simulink model "SAD_project"  (R2023b)
settings: Solver=ode4  StartTime=t0  StopTime=tf  FixedStep=t_step  RelTol=1e-3
values from neighbouring files (symbols this model uses):
  A = 1e-2.*[6, 6, 6, 6, 4, 4, 12, 12, 12, 12]'    [SAD_project_code.m]
  A1 = ones(length(BODY),1)    [SAD_project_code.m]
  BODY = [1, 0, 0 ... (first row only)    [SAD_project_code.m]
  c = 3e8    (= 300000000)    [SAD_project_code.m]
  DCM_eci_per = rotationMatrix(rad2deg(i),rad2deg(OM), rad2deg(om))    [SAD_project_code.m]
  e = 0.001    [SAD_project_code.m]
  epsilon = deg2rad(23.45)    [SAD_project_code.m]
  Fe = 1358    [SAD_project_code.m]
  FS = 800e-9    (= 8e-07)    [SAD_project_code.m]
  H0 = 1e-9.*[-29404.8 -1450.9 4652.5]'    [SAD_project_code.m]
  i = deg2rad(60)    [SAD_project_code.m]
  I = [Ix, 0, 0; 0, Iy, 0; 0, 0, Iz]    [SAD_project_code.m]
  I_inv = inv(I)    [SAD_project_code.m]
  inc_tot = sqrt(inc_lin^2 + inc_acc^2)    [SAD_project_code.m]
  j_b = [0.01 0.05 0.01]'    [SAD_project_code.m]
  MJD2000_initial = date2mjd2000(date0)    [SAD_project_code.m]
  mu_E = astroConstants(13)    [SAD_project_code.m]
  n_e = sqrt(mu_E/a^3)    [SAD_project_code.m]
  p = a*(1-e^2)    [SAD_project_code.m]
  pd = 0.1.*A1    [SAD_project_code.m]
  ps = [0.5, 0.5, 0.5, 0.5, 0.5, 0.5, 0.1, 0.1, 0.1, 0.1]'    [SAD_project_code.m]
  q0 = [0 0 0 1]    [SAD_project_code.m]
  r1 = r(:,1) + CMC_position(1).*ones(10,1)    [SAD_project_code.m]
  r2 = r(:,2) + CMC_position(2).*ones(10,1)    [SAD_project_code.m]
  r3 = r(:,3)+ CMC_position(3).*ones(10,1)    [SAD_project_code.m]
  R_E = astroConstants(23)    [SAD_project_code.m]
  th0 = deg2rad(0)    [SAD_project_code.m]
  ts_sensor = t_step    (= 0.01)    [SAD_project_code.m]
  w0 = [wx0 wy0 wz0]'    [SAD_project_code.m]
  w_E = deg2rad(15.04)/60/60    [SAD_project_code.m]
  w_r = 0    [SAD_project_code.m]
libraries: matrix_library x6, simulink x1
settings Model: Creator=samue  LastModifiedBy=samue

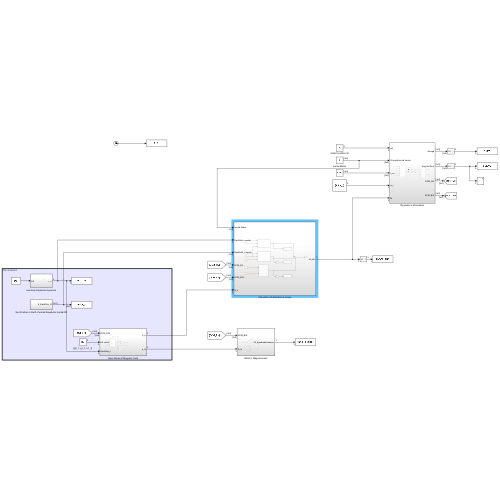
[thumbnail: Simulink's stored preview of the top-level diagram]
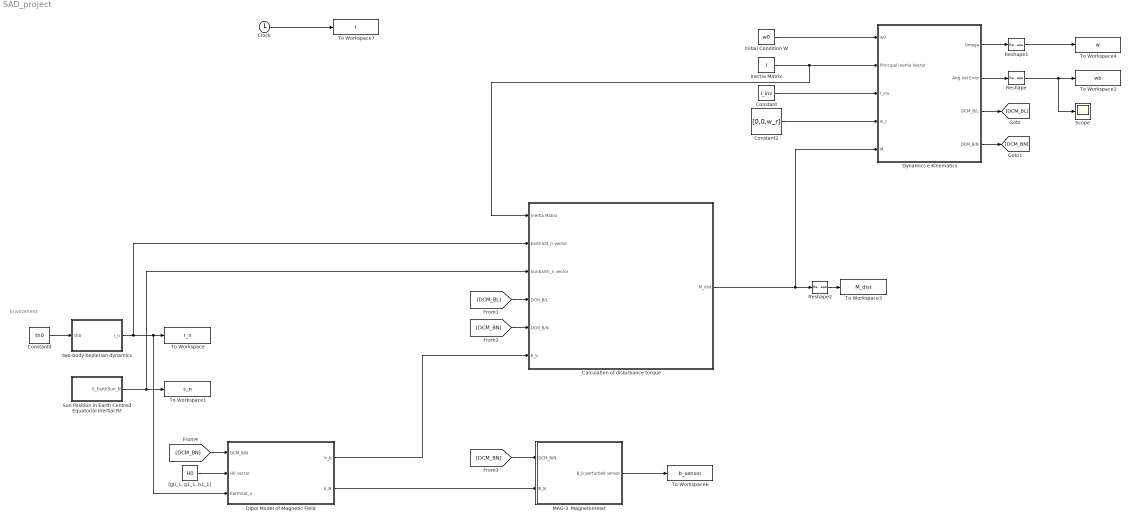
== system SAD_project ==
  note: Enviroment
  Calculation of disturbance torque : Subsystem
  Clock : Clock
  Constant : Constant  Value=I_inv
  Constant2 : Constant  Value=[0,0,w_r]
  Constant4 : Constant  Value=th0
  Dipol Model of Magnetic Field : Subsystem
  Dynamics e Kinematics : Subsystem
  Inertia Matrix : Constant  Value=I  VectorParams1D=off
  Initial Condition W : Constant  Value=w0
  MAG-3  Magnetometer : Subsystem
  Reshape : Reshape
  Reshape1 : Reshape
  Reshape2 : Reshape
  Scope : Scope
  Sun Position in Earth Centred Equatorial Inertial RF : Subsystem
  To Workspace : ToWorkspace  VariableName=r_n  SampleTime=-1
  To Workspace1 : ToWorkspace  VariableName=s_n  SampleTime=-1
  To Workspace2 : ToWorkspace  VariableName=wb  SampleTime=-1
  To Workspace3 : ToWorkspace  VariableName=M_dist  SaveFormat=Timeseries  SampleTime=-1
  To Workspace4 : ToWorkspace  VariableName=w  SampleTime=-1
  To Workspace6 : ToWorkspace  VariableName=b_sensor  SampleTime=-1
  To Workspace7 : ToWorkspace  VariableName=t  SampleTime=-1
  "[g0_1, g1_1, h1_1]" : Constant  Value=H0
  two-body Keplerian dynamics : Subsystem
  wires:
  two-body Keplerian dynamics/1(r_n) -> Calculation of disturbance torque/2(EarthSat_n vector), To Workspace/1, Dipol Model of Magnetic Field/3(EarthSat_n)
  Inertia Matrix/1 -> Calculation of disturbance torque/1(Inertia Matrix), Dynamics e Kinematics/2("Principal Inertia Vector ")
  Initial Condition W/1 -> Dynamics e Kinematics/1(w0)
  Reshape/1 -> Scope/1, To Workspace2/1
  Dynamics e Kinematics/2(Ang Vel Error) -> Reshape/1
  Dynamics e Kinematics/3(DCM_B/L) -> [DCM_BL]
  Dynamics e Kinematics/1(Omega) -> Reshape1/1
  Sun Position in Earth Centred Equatorial Inertial RF/1(S_EarthSun_N) -> To Workspace1/1, Calculation of disturbance torque/3(SunEarth_n vector)
  Constant2/1 -> Dynamics e Kinematics/4(w_r)
  Constant4/1 -> two-body Keplerian dynamics/1(th0)
  Constant/1 -> Dynamics e Kinematics/3(I_inv)
  Clock/1 -> To Workspace7/1
  Dynamics e Kinematics/4(DCM_B/N) -> [DCM_BN]
  Calculation of disturbance torque/1(M_dist) -> Reshape2/1, Dynamics e Kinematics/5(M)
  "[g0_1, g1_1, h1_1]"/1 -> Dipol Model of Magnetic Field/2(H0 vector)
  Dipol Model of Magnetic Field/1(b_b) -> Calculation of disturbance torque/6(B_b)
  MAG-3  Magnetometer/1(B_b perturbed sensor) -> To Workspace6/1
  [DCM_BN] -> MAG-3  Magnetometer/1(DCM_B/N)
  [DCM_BL] -> Calculation of disturbance torque/4(DCM_B/L)
  [DCM_BN] -> Calculation of disturbance torque/5(DCM_B/N)
  [DCM_BN] -> Dipol Model of Magnetic Field/1(DCM_B/N)
  Dipol Model of Magnetic Field/2(b_N) -> MAG-3  Magnetometer/2(B_N)
  Reshape1/1 -> To Workspace4/1
  Reshape2/1 -> To Workspace3/1

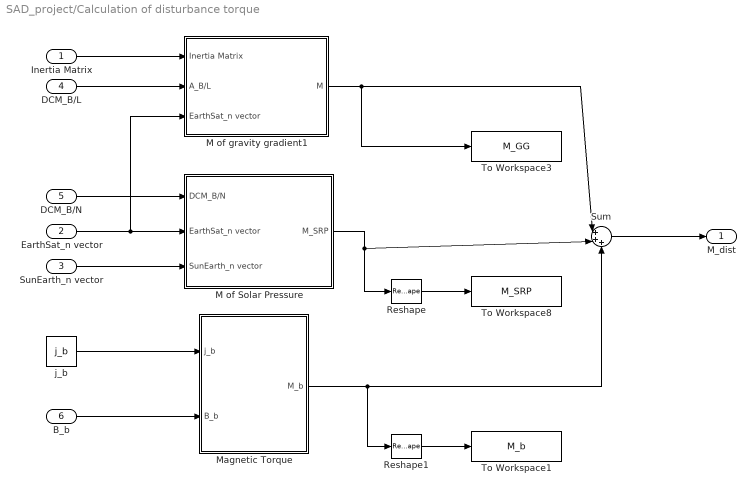
== system SAD_project/Calculation of disturbance torque ==
  Inertia Matrix : Inport
  EarthSat_n vector : Inport  Port=2
  SunEarth_n vector : Inport  Port=3
  DCM_B/L : Inport  Port=4
  DCM_B/N : Inport  Port=5
  B_b : Inport  Port=6
  M of Solar Pressure : Subsystem
  M of gravity gradient1 : Subsystem
  Magnetic Torque : Subsystem
  Reshape : Reshape
  Reshape1 : Reshape
  Sum : Sum  Inputs=|+++
  To Workspace1 : ToWorkspace  VariableName=M_b  SampleTime=-1
  To Workspace3 : ToWorkspace  VariableName=M_GG  SampleTime=-1
  To Workspace8 : ToWorkspace  VariableName=M_SRP  SampleTime=-1
  j_b : Constant  Value=j_b
  M_dist : Outport
  wires:
  DCM_B/L/1 -> M of gravity gradient1/2(A_B/L)
  j_b/1 -> Magnetic Torque/1(j_b)
  Magnetic Torque/1(M_b) -> Sum/3, Reshape1/1
  B_b/1 -> Magnetic Torque/2(B_b)
  Inertia Matrix/1 -> M of gravity gradient1/1(Inertia Matrix)
  M of Solar Pressure/1(M_SRP) -> Sum/2, Reshape/1
  EarthSat_n vector/1 -> M of gravity gradient1/3(EarthSat_n vector), M of Solar Pressure/2(EarthSat_n vector)
  DCM_B/N/1 -> M of Solar Pressure/1(DCM_B/N)
  SunEarth_n vector/1 -> M of Solar Pressure/3(SunEarth_n vector)
  Sum/1 -> M_dist/1
  Reshape/1 -> To Workspace8/1
  Reshape1/1 -> To Workspace1/1
  M of gravity gradient1/1(M) -> To Workspace3/1, Sum/1

== system SAD_project/Dipol Model of Magnetic Field ==
  note: CODE TO ADD
      | % Definition of Magnetic Field (Dipole model)
      |  j_b = [0.01 0.05 0.01]';
      | H0 = 1e-9.*[-29404.8 -1450.9 4652.5]';
  DCM_B/N : Inport
  H0 vector : Inport  Port=2
  EarthSat_n : Inport  Port=3
  Calculation of b_n : Subsystem
  Matrix Multiply : Product  Multiplication=Matrix(*)
  To Workspace : ToWorkspace  VariableName=bn  SampleTime=-1
  b_b : Outport
  b_N : Outport  Port=2
  wires:
  Matrix Multiply/1 -> b_b/1
  DCM_B/N/1 -> Matrix Multiply/1
  H0 vector/1 -> Calculation of b_n/1(H0 vector)
  EarthSat_n/1 -> Calculation of b_n/2(EarthSat_n)
  Calculation of b_n/1(b_N) -> To Workspace/1, b_N/1, Matrix Multiply/2

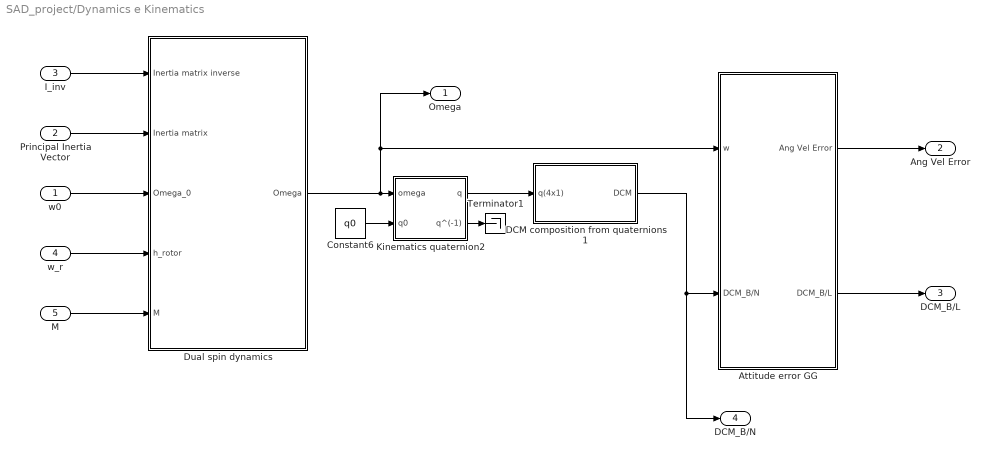
== system SAD_project/Dynamics e Kinematics ==
  w0 : Inport
  "Principal Inertia Vector " : Inport  Port=2
  I_inv : Inport  Port=3
  w_r : Inport  Port=4
  M : Inport  Port=5
  Attitude error GG : Subsystem
  Constant6 : Constant  Value=q0
  DCM composition from quaternions 1 : Subsystem  AncestorBlock=LibrarySAD5/DCM composition from quaternions
  Dual spin dynamics : Subsystem  AncestorBlock=LibrarySAD5/Dual spin dynamics
  Kinematics quaternion2 : Subsystem
  Terminator1 : Terminator
  Omega : Outport
  Ang Vel Error : Outport  Port=2
  DCM_B/L : Outport  Port=3
  DCM_B/N : Outport  Port=4
  wires:
  DCM composition from quaternions 1/1(DCM) -> DCM_B/N/1, Attitude error GG/2(DCM_B/N)
  Constant6/1 -> Kinematics quaternion2/2(q0)
  Dual spin dynamics/1(Omega) -> Omega/1, Attitude error GG/1(w), Kinematics quaternion2/1(omega)
  Kinematics quaternion2/2(q^(-1)) -> Terminator1/1
  M/1 -> Dual spin dynamics/5(M)
  w0/1 -> Dual spin dynamics/3(Omega_0)
  "Principal Inertia Vector "/1 -> Dual spin dynamics/2(Inertia matrix)
  Kinematics quaternion2/1(q) -> DCM composition from quaternions 1/1(q(4x1))
  Attitude error GG/2(DCM_B/L) -> DCM_B/L/1
  Attitude error GG/1(Ang Vel Error) -> Ang Vel Error/1
  I_inv/1 -> Dual spin dynamics/1(Inertia matrix inverse)
  w_r/1 -> Dual spin dynamics/4(h_rotor)

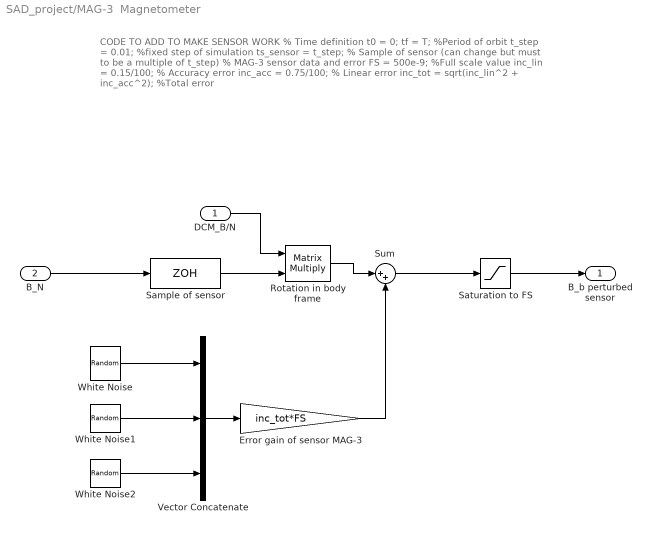
== system SAD_project/MAG-3  Magnetometer ==
  note: CODE TO ADD TO MAKE SENSOR WORK
      | % Time definition
      | t0 = 0;
      | tf = T; %Period of orbit
      | t_step = 0.01; %fixed step of simulation
      | ts_sensor = t_step; % Sample of sensor (can change but must to be a multiple of t_step)
      |
      | % MAG-3 sensor data and error
      | FS = 500e-9; %Full scale value
      | inc_lin = 0.15/100; % Accuracy error
      | inc_acc = 0.75/100; % Linear error
      | inc_tot = sqrt(inc_lin^2 + inc_acc^2); %Total error
  DCM_B/N : Inport
  B_N : Inport  Port=2
  Error gain of sensor MAG-3 : Gain  Gain=inc_tot*FS
  Rotation in body frame : Product  Multiplication=Matrix(*)
  Sample of sensor : ZeroOrderHold  SampleTime=ts_sensor
  Saturation to FS : Saturate  UpperLimit=FS  LowerLimit=-FS
  Sum : Sum  Inputs=|++
  Vector Concatenate : Concatenate  NumInputs=3
  White Noise : RandomNumber  DisableCoverage=on  Seed=1  SampleTime=ts_sensor
  White Noise1 : RandomNumber  DisableCoverage=on  Seed=2  SampleTime=ts_sensor
  White Noise2 : RandomNumber  DisableCoverage=on  Seed=3  SampleTime=ts_sensor
  B_b perturbed sensor : Outport
  wires:
  Vector Concatenate/1 -> Error gain of sensor MAG-3/1
  White Noise/1 -> Vector Concatenate/1
  Error gain of sensor MAG-3/1 -> Sum/2
  White Noise2/1 -> Vector Concatenate/3
  White Noise1/1 -> Vector Concatenate/2
  Sum/1 -> Saturation to FS/1
  B_N/1 -> Sample of sensor/1
  DCM_B/N/1 -> Rotation in body frame/1
  Saturation to FS/1 -> B_b perturbed sensor/1
  Sample of sensor/1 -> Rotation in body frame/2
  Rotation in body frame/1 -> Sum/1

== system SAD_project/Sun Position in Earth Centred Equatorial Inertial RF ==
  1 day in second1 : Constant  Value=3600*24
  Clock1 : Clock
  Constant2 : Constant  Value=MJD2000_initial
  Constant3 : Constant  Value=[1 0 0; 0 cos(epsilon) -sin(epsilon); 0 sin(epsilon) cos(epsilon)]
  Divide1 : Product  Inputs=*/
  Gain1 : Gain  Gain=-1
  MATLAB Function1 : MATLAB Function  TreatAsAtomicUnit=on
  Matrix Multiply1 : Product  Multiplication=Matrix(*)
  Sum1 : Sum  Inputs=|++
  S_EarthSun_N : Outport
  wires:
  1 day in second1/1 -> Divide1/2
  Sum1/1 -> MATLAB Function1/1(MJD2000)  "mjd2000"
  Divide1/1 -> Sum1/1
  Constant3/1 -> Matrix Multiply1/1
  Matrix Multiply1/1 -> Gain1/1
  Clock1/1 -> Divide1/1
  MATLAB Function1/1(r) -> Matrix Multiply1/2
  Constant2/1 -> Sum1/2
  Gain1/1 -> S_EarthSun_N/1

== system SAD_project/two-body Keplerian dynamics ==
  th0 : Inport
  Constant : Constant  Value=DCM_eci_per
  Integretion of true anomaly : Subsystem
  Matrix Multiply : Product  Multiplication=Matrix(*)
  Transpose : Math  Operator=transpose
  r_perifocal : Subsystem
  r_n : Outport
  wires:
  th0/1 -> Integretion of true anomaly/1(th0)
  Integretion of true anomaly/1(th) -> r_perifocal/1(th)
  Constant/1 -> Transpose/1
  Transpose/1 -> Matrix Multiply/1
  r_perifocal/1(r_per) -> Matrix Multiply/2
  Matrix Multiply/1 -> r_n/1

== system SAD_project/Calculation of disturbance torque/M of Solar Pressure ==
  DCM_B/N : Inport
  EarthSat_n vector : Inport  Port=2
  SunEarth_n vector : Inport  Port=3
  Calculation of F_i : Subsystem
  Constant : Constant  Value=BODY
  Matrix Multiply : Product  Multiplication=Matrix(*)
  Normalize Vector : Subsystem
  Subtract : Sum  Inputs=--
  Torque calculation : Subsystem
  M_SRP : Outport
  wires:
  Calculation of F_i/1(F_i matrix) -> Torque calculation/1(F_i Matrix)
  EarthSat_n vector/1 -> Subtract/1
  Constant/1 -> Calculation of F_i/1(body versor matrix)
  Normalize Vector/1(Versor) -> Calculation of F_i/2(Sb_vector1)
  Torque calculation/1(M_SRP) -> M_SRP/1
  SunEarth_n vector/1 -> Subtract/2
  Subtract/1 -> Matrix Multiply/2  "SatSun_vector inertial"
  Matrix Multiply/1 -> Normalize Vector/1(Vector)
  DCM_B/N/1 -> Matrix Multiply/1

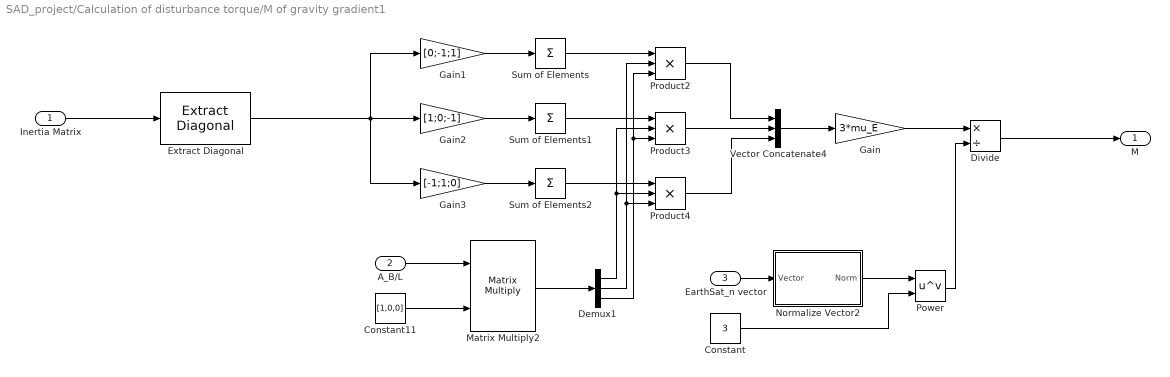
== system SAD_project/Calculation of disturbance torque/M of gravity gradient1 ==
  Inertia Matrix : Inport
  A_B/L : Inport  Port=2
  EarthSat_n vector : Inport  Port=3
  Constant : Constant  Value=3
  Constant11 : Constant  Value=[1,0,0]
  Demux1 : Demux  Outputs=3
  Divide : Product  Inputs=*/
  Extract Diagonal : matrix_library/Extract Diagonal
      settings: LibrarySourceBlock=|
      | simulink/Matrix
      | Operations/Extract Diagonal
  Gain : Gain  Gain=3*mu_E
  Gain1 : Gain  Gain=[0;-1;1]
  Gain2 : Gain  Gain=[1;0;-1]
  Gain3 : Gain  Gain=[-1;1;0]
  Matrix Multiply2 : Product  Multiplication=Matrix(*)
  Normalize Vector2 : Subsystem  AncestorBlock=LibrarySAD5/Normalize Vector1
  Power : Math  Operator=pow
  Product2 : Product  Inputs=3
  Product3 : Product  Inputs=3
  Product4 : Product  Inputs=3
  Sum of Elements : Sum  Inputs=+
  Sum of Elements1 : Sum  Inputs=+
  Sum of Elements2 : Sum  Inputs=+
  Vector Concatenate4 : Concatenate  NumInputs=3
  M : Outport
  wires:
  Demux1/3 -> Product2/3, Product3/3
  Product2/1 -> Vector Concatenate4/1
  Matrix Multiply2/1 -> Demux1/1
  Product4/1 -> Vector Concatenate4/3
  Product3/1 -> Vector Concatenate4/2
  Demux1/1 -> Product4/2, Product3/2
  Constant11/1 -> Matrix Multiply2/2
  Demux1/2 -> Product4/3, Product2/2
  A_B/L/1 -> Matrix Multiply2/1
  Vector Concatenate4/1 -> Gain/1
  Gain1/1 -> Sum of Elements/1
  Gain2/1 -> Sum of Elements1/1
  Gain3/1 -> Sum of Elements2/1
  Sum of Elements/1 -> Product2/1
  Sum of Elements1/1 -> Product3/1
  Sum of Elements2/1 -> Product4/1
  Inertia Matrix/1 -> Extract Diagonal/1
  Gain/1 -> Divide/1
  EarthSat_n vector/1 -> Normalize Vector2/1(Vector)
  Power/1 -> Divide/2
  Constant/1 -> Power/2
  Normalize Vector2/1(Norm) -> Power/1
  Divide/1 -> M/1
  Extract Diagonal/1 -> Gain1/1, Gain2/1, Gain3/1

== system SAD_project/Calculation of disturbance torque/Magnetic Torque ==
  j_b : Inport
  B_b : Inport  Port=2
  Cross Product : matrix_library/Cross Product
  M_b : Outport
  wires:
  Cross Product/1 -> M_b/1
  j_b/1 -> Cross Product/1
  B_b/1 -> Cross Product/2

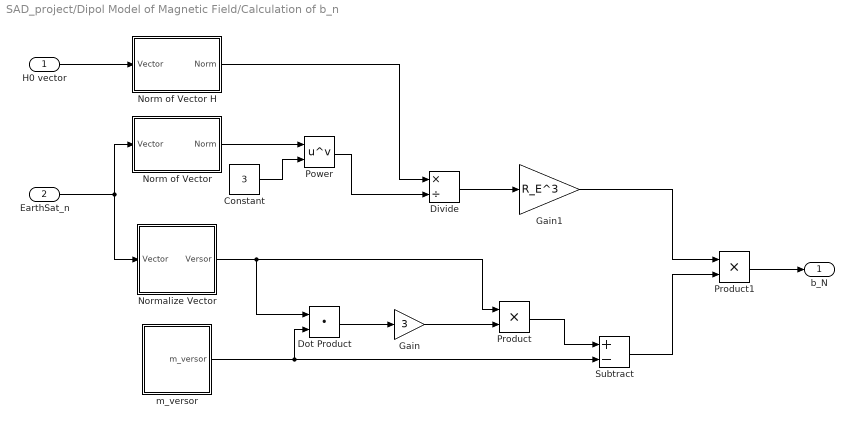
== system SAD_project/Dipol Model of Magnetic Field/Calculation of b_n ==
  H0 vector : Inport
  EarthSat_n : Inport  Port=2
  Constant : Constant  Value=3
  Divide : Product  Inputs=*/
  Dot Product : DotProduct  OutDataTypeStr=Inherit: Inherit via internal rule
  Gain : Gain  Gain=3
  Gain1 : Gain  Gain=R_E^3
  Norm of Vector : Subsystem  AncestorBlock=LibrarySAD5/Normalize Vector1
  Norm of Vector H : Subsystem  AncestorBlock=LibrarySAD5/Normalize Vector1
  Normalize Vector : Subsystem
  Power : Math  Operator=pow
  Product : Product
  Product1 : Product
  Subtract : Sum  Inputs=+-
  m_versor : Subsystem
  b_N : Outport
  wires:
  Norm of Vector/1(Norm) -> Power/1
  Product/1 -> Subtract/1
  Divide/1 -> Gain1/1
  EarthSat_n/1 -> Norm of Vector/1(Vector), Normalize Vector/1(Vector)
  Normalize Vector/1(Versor) -> Product/1, Dot Product/1
  Gain1/1 -> Product1/1
  m_versor/1(m_versor) -> Dot Product/2, Subtract/2
  Gain/1 -> Product/2
  Product1/1 -> b_N/1
  Constant/1 -> Power/2
  Dot Product/1 -> Gain/1
  Subtract/1 -> Product1/2
  Norm of Vector H/1(Norm) -> Divide/1
  Power/1 -> Divide/2
  H0 vector/1 -> Norm of Vector H/1(Vector)

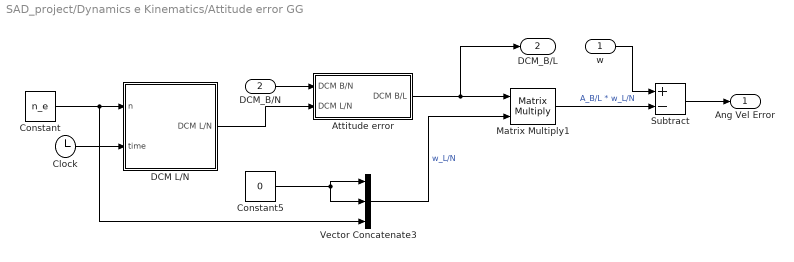
== system SAD_project/Dynamics e Kinematics/Attitude error GG ==
  w : Inport
  DCM_B/N : Inport  Port=2
  Attitude error : Subsystem
  Clock : Clock
  Constant : Constant  Value=n_e
  Constant5 : Constant  Value=0
  DCM L/N : Subsystem
  Matrix Multiply1 : Product  Multiplication=Matrix(*)
  Subtract : Sum  Inputs=+-
  Vector Concatenate3 : Concatenate  NumInputs=3
  Ang Vel Error : Outport
  DCM_B/L : Outport  Port=2
  wires:
  Clock/1 -> DCM L/N/2(time)
  Constant5/1 -> Vector Concatenate3/2, Vector Concatenate3/1
  Vector Concatenate3/1 -> Matrix Multiply1/2  "w_L/N"
  DCM_B/N/1 -> Attitude error/1(DCM B/N)
  DCM L/N/1(DCM L/N) -> Attitude error/2(DCM L/N)
  Attitude error/1(DCM B/L) -> Matrix Multiply1/1, DCM_B/L/1
  Matrix Multiply1/1 -> Subtract/2  "A_B/L * w_L/N"
  w/1 -> Subtract/1
  Subtract/1 -> Ang Vel Error/1
  Constant/1 -> DCM L/N/1(n), Vector Concatenate3/3

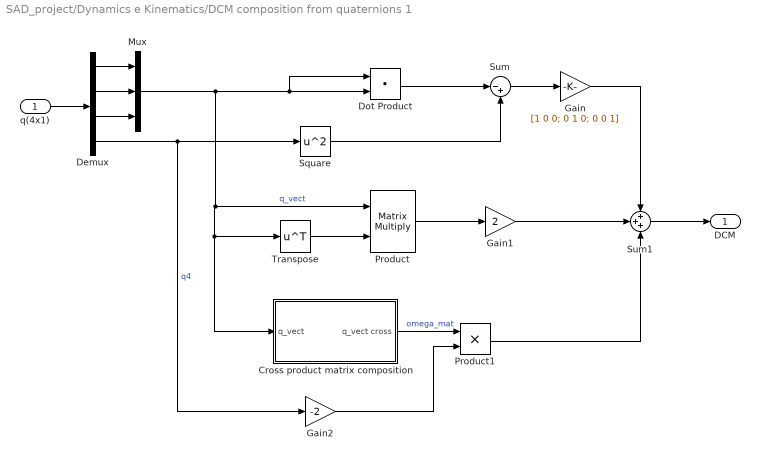
== system SAD_project/Dynamics e Kinematics/DCM composition from quaternions 1 ==
  q(4x1) : Inport
  Cross product matrix composition : Subsystem
  Demux : Demux
  Dot Product : DotProduct  OutDataTypeStr=Inherit: Inherit via internal rule
  Gain : Gain  Gain=[1 0 0; 0 1 0; 0 0 1]
  Gain1 : Gain  Gain=2
  Gain2 : Gain  Gain=-2
  Mux : Mux  Inputs=3
  Product : Product  Multiplication=Matrix(*)
  Product1 : Product
  Square : Math  Operator=square
  Sum : Sum  Inputs=|-+
  Sum1 : Sum  Inputs=+++
  Transpose : Math  Operator=transpose
  DCM : Outport
  wires:
  Gain/1 -> Sum1/1
  Demux/1 -> Mux/1
  q(4x1)/1 -> Demux/1
  Demux/2 -> Mux/2
  Mux/1 -> Dot Product/2, Dot Product/1, Product/1, Cross product matrix composition/1(q_vect), Transpose/1  "q_vect"
  Demux/4 -> Gain2/1, Square/1  "q4"
  Demux/3 -> Mux/3
  Dot Product/1 -> Sum/1
  Sum/1 -> Gain/1
  Square/1 -> Sum/2
  Transpose/1 -> Product/2
  Product/1 -> Gain1/1
  Gain2/1 -> Product1/2
  Cross product matrix composition/1(q_vect cross) -> Product1/1  "omega_mat"
  Product1/1 -> Sum1/3
  Gain1/1 -> Sum1/2
  Sum1/1 -> DCM/1

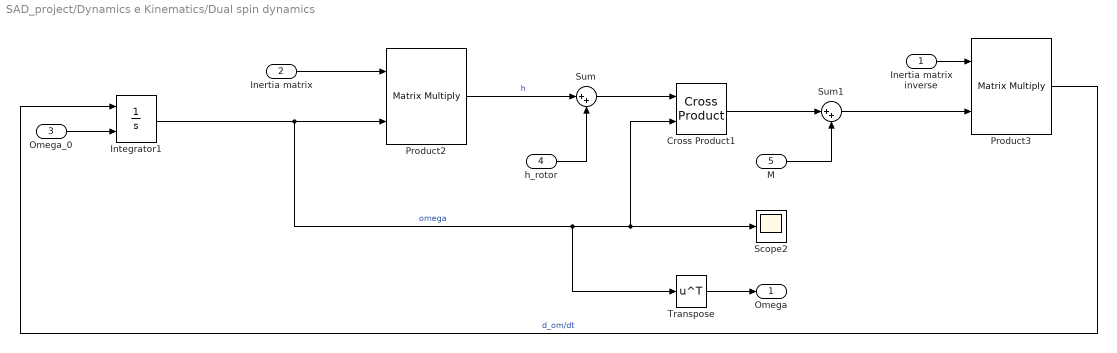
== system SAD_project/Dynamics e Kinematics/Dual spin dynamics ==
  Inertia matrix inverse : Inport
  Inertia matrix : Inport  Port=2
  Omega_0 : Inport  Port=3
  h_rotor : Inport  Port=4
  M : Inport  Port=5
  Cross Product1 : matrix_library/Cross Product
  Integrator1 : Integrator  InitialConditionSource=external
  Product2 : Product  Multiplication=Matrix(*)
  Product3 : Product  Multiplication=Matrix(*)
  Scope2 : Scope
  Sum : Sum  Inputs=|++
  Sum1 : Sum  Inputs=|++
  Transpose : Math  Operator=transpose
  Omega : Outport
  wires:
  M/1 -> Sum1/2
  Sum1/1 -> Product3/2
  Omega_0/1 -> Integrator1/2
  Product2/1 -> Sum/1  "h"
  Inertia matrix/1 -> Product2/1
  Product3/1 -> Integrator1/1  "d_om/dt"
  h_rotor/1 -> Sum/2
  Integrator1/1 -> Product2/2, Cross Product1/2, Scope2/1, Transpose/1  "omega"
  Cross Product1/1 -> Sum1/1
  Inertia matrix inverse/1 -> Product3/1
  Sum/1 -> Cross Product1/1
  Transpose/1 -> Omega/1

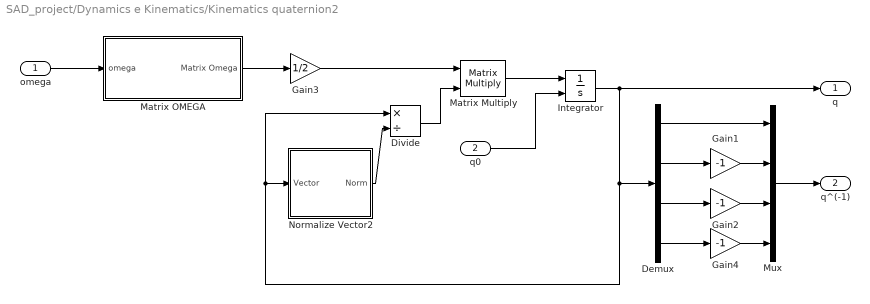
== system SAD_project/Dynamics e Kinematics/Kinematics quaternion2 ==
  omega : Inport
  q0 : Inport  Port=2
  Demux : Demux
  Divide : Product  Inputs=*/
  Gain1 : Gain  Gain=-1
  Gain2 : Gain  Gain=-1
  Gain3 : Gain  Gain=1/2
  Gain4 : Gain  Gain=-1
  Integrator : Integrator  InitialConditionSource=external
  Matrix Multiply : Product  Multiplication=Matrix(*)
  Matrix OMEGA : Subsystem
  Mux : Mux
  Normalize Vector2 : Subsystem
  q : Outport
  q^(-1) : Outport  Port=2
  wires:
  Gain3/1 -> Matrix Multiply/1
  Matrix Multiply/1 -> Integrator/1
  omega/1 -> Matrix OMEGA/1(omega)
  Integrator/1 -> Normalize Vector2/1(Vector), Divide/1, Demux/1, q/1
  Matrix OMEGA/1(Matrix Omega) -> Gain3/1
  q0/1 -> Integrator/2
  Demux/2 -> Gain1/1
  Demux/3 -> Gain2/1
  Demux/4 -> Gain4/1
  Gain1/1 -> Mux/2
  Gain2/1 -> Mux/3
  Gain4/1 -> Mux/4
  Demux/1 -> Mux/1
  Mux/1 -> q^(-1)/1
  Normalize Vector2/1(Norm) -> Divide/2
  Divide/1 -> Matrix Multiply/2

== system SAD_project/two-body Keplerian dynamics/Integretion of true anomaly ==
  th0 : Inport
  (1-e^2)^(3/2) : Subsystem
  Constant : Constant
  Cos : Trigonometry  Operator=cos
  Divide : Product  Inputs=*/
  Gain : Gain  Gain=e
  Gain1 : Gain  Gain=n_e
  Integrator : Integrator  InitialConditionSource=external
  Product : Product
  Sum : Sum  Inputs=|++
  th : Outport
  wires:
  Sum/1 -> Product/1, Product/2
  Integrator/1 -> th/1, Cos/1  "theta"
  Divide/1 -> Integrator/1
  Constant/1 -> Sum/1
  Product/1 -> Gain1/1
  Cos/1 -> Gain/1
  Gain/1 -> Sum/2
  (1-e^2)^(3/2)/1(Out1) -> Divide/2
  th0/1 -> Integrator/2
  Gain1/1 -> Divide/1

== system SAD_project/two-body Keplerian dynamics/r_perifocal ==
  th : Inport
  Calculation of norm r : Subsystem
  Constant : Constant  Value=0
  Cos : Trigonometry  Operator=cos
  Mux : Mux  Inputs=3
  Product : Product
  Sin : Trigonometry
  r_per : Outport
  wires:
  Constant/1 -> Mux/3
  Cos/1 -> Mux/1
  th/1 -> Calculation of norm r/1(th), Cos/1, Sin/1
  Sin/1 -> Mux/2
  Mux/1 -> Product/1  "r_n"
  Calculation of norm r/1(Norm(r)) -> Product/2
  Product/1 -> r_per/1  "r_n"

== system SAD_project/Calculation of disturbance torque/M of Solar Pressure/Calculation of F_i ==
  body versor matrix : Inport
  Sb_vector1 : Inport  Port=2
  (1-ps)*Sb + (2ps*dot(SB,Nb) +2/3pd))*Ni : Subsystem
  Constant1 : Constant  Value=A
  Eliminate effect of face in shadow : Subsystem
  Matrix Concatenate1 : Concatenate  NumInputs=3  Mode=Multidimensional array  ConcatenateDimension=2
  Matrix Multiply1 : Product
  Subsystem : Subsystem
  dot(Sb,Nb) : Subsystem
  F_i matrix : Outport
  wires:
  dot(Sb,Nb)/1(dot(SB,Nb)) -> (1-ps)*Sb + (2ps*dot(SB,Nb) +2/3pd))*Ni/2(dot(Sb,Nb)), Eliminate effect of face in shadow/1(dot(SB,Nb))
  Sb_vector1/1 -> dot(Sb,Nb)/2(Sb_vector1)
  Subsystem/1(-PA*dot(SB,Nb)) -> Matrix Concatenate1/3, Matrix Concatenate1/1, Matrix Concatenate1/2
  (1-ps)*Sb + (2ps*dot(SB,Nb) +2/3pd))*Ni/1(Out1) -> Matrix Multiply1/2
  Constant1/1 -> Subsystem/2(A)
  Matrix Concatenate1/1 -> Matrix Multiply1/1  "matrix of -PA*dot(SB,Nb)"
  Matrix Multiply1/1 -> F_i matrix/1
  body versor matrix/1 -> (1-ps)*Sb + (2ps*dot(SB,Nb) +2/3pd))*Ni/1(body), dot(Sb,Nb)/1(body versor matrix)
  dot(Sb,Nb)/2(Sb_matrix) -> (1-ps)*Sb + (2ps*dot(SB,Nb) +2/3pd))*Ni/3(Sb versor)
  Eliminate effect of face in shadow/1(dot(SB,Nb)-clean) -> Subsystem/1(dot(SB,Nb))

== system SAD_project/Calculation of disturbance torque/M of Solar Pressure/Normalize Vector ==
  Vector : Inport
  Divide : Product  Inputs=*/
  Normalize Vector : Subsystem  AncestorBlock=LibrarySAD5/Normalize Vector1
  Versor : Outport
  wires:
  Vector/1 -> Normalize Vector/1(Vector), Divide/1
  Divide/1 -> Versor/1
  Normalize Vector/1(Norm) -> Divide/2

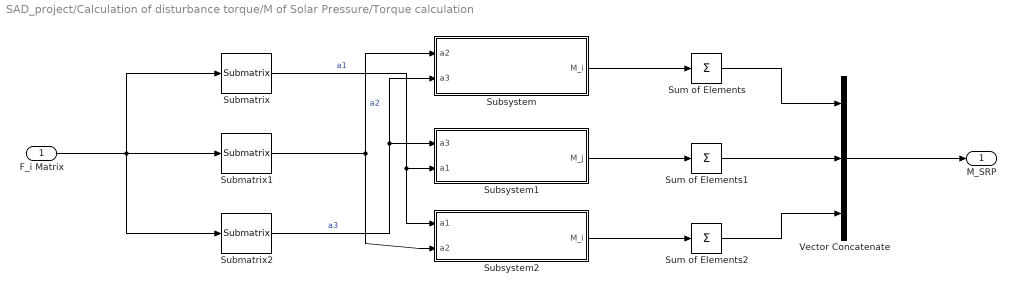
== system SAD_project/Calculation of disturbance torque/M of Solar Pressure/Torque calculation ==
  F_i Matrix : Inport
  Submatrix : matrix_library/Submatrix  RowSpan=All rows  RowStartMode=First  RowStartIndex=1  RowEndMode=Last  RowEndIndex=1  ColSpan=One column  ColStartMode=First  ColStartIndex=1  ColEndMode=Last  ColEndIndex=1
  Submatrix1 : matrix_library/Submatrix  RowSpan=All rows  RowStartMode=First  RowStartIndex=1  RowEndMode=Last  RowEndIndex=1  ColSpan=One column  ColStartMode=Index  ColStartIndex=2  ColEndMode=Last  ColEndIndex=1
  Submatrix2 : matrix_library/Submatrix  RowSpan=All rows  RowStartMode=First  RowStartIndex=1  RowEndMode=Last  RowEndIndex=1  ColSpan=One column  ColStartMode=Last  ColStartIndex=1  ColEndMode=Last  ColEndIndex=1
  Subsystem : Subsystem
  Subsystem1 : Subsystem
  Subsystem2 : Subsystem
  Sum of Elements : Sum  Inputs=+
  Sum of Elements1 : Sum  Inputs=+
  Sum of Elements2 : Sum  Inputs=+
  Vector Concatenate : Concatenate  NumInputs=3
  M_SRP : Outport
  wires:
  Subsystem/1(M_i) -> Sum of Elements/1
  Submatrix2/1 -> Subsystem1/1(a3), Subsystem/2(a3)  "a3"
  Subsystem2/1(M_i) -> Sum of Elements2/1
  Submatrix1/1 -> Subsystem2/2(a2), Subsystem/1(a2)  "a2"
  Subsystem1/1(M_j) -> Sum of Elements1/1
  Submatrix/1 -> Subsystem1/2(a1), Subsystem2/1(a1)  "a1"
  F_i Matrix/1 -> Submatrix/1, Submatrix2/1, Submatrix1/1
  Sum of Elements/1 -> Vector Concatenate/1
  Sum of Elements1/1 -> Vector Concatenate/2
  Sum of Elements2/1 -> Vector Concatenate/3
  Vector Concatenate/1 -> M_SRP/1

== system SAD_project/Calculation of disturbance torque/M of gravity gradient1/Normalize Vector2 ==
  Vector : Inport
  Dot Product : DotProduct  OutDataTypeStr=Inherit: Inherit via internal rule
  Sqrt : Sqrt
  Norm : Outport
  wires:
  Sqrt/1 -> Norm/1
  Vector/1 -> Dot Product/1, Dot Product/2
  Dot Product/1 -> Sqrt/1

== system SAD_project/Dipol Model of Magnetic Field/Calculation of b_n/Norm of Vector ==
  Vector : Inport
  Dot Product : DotProduct  OutDataTypeStr=Inherit: Inherit via internal rule
  Sqrt : Sqrt
  Norm : Outport
  wires:
  Sqrt/1 -> Norm/1
  Vector/1 -> Dot Product/1, Dot Product/2
  Dot Product/1 -> Sqrt/1

== system SAD_project/Dipol Model of Magnetic Field/Calculation of b_n/Norm of Vector H ==
  Vector : Inport
  Dot Product : DotProduct  OutDataTypeStr=Inherit: Inherit via internal rule
  Sqrt : Sqrt
  Norm : Outport
  wires:
  Sqrt/1 -> Norm/1
  Vector/1 -> Dot Product/1, Dot Product/2
  Dot Product/1 -> Sqrt/1

== system SAD_project/Dipol Model of Magnetic Field/Calculation of b_n/Normalize Vector ==
  Vector : Inport
  Divide : Product  Inputs=*/
  Normalize Vector1 : Subsystem  AncestorBlock=LibrarySAD5/Normalize Vector1
  Versor : Outport
  wires:
  Vector/1 -> Normalize Vector1/1(Vector), Divide/1
  Divide/1 -> Versor/1
  Normalize Vector1/1(Norm) -> Divide/2

== system SAD_project/Dipol Model of Magnetic Field/Calculation of b_n/m_versor ==
  Clock : Clock
  Constant : Constant  Value=cos(deg2rad(11.5))
  Cos : Trigonometry  Operator=cos
  Gain : Gain  Gain=deg2rad(w_E)
  Gain1 : Gain  Gain=sin(deg2rad(11.5))
  Gain2 : Gain  Gain=sin(deg2rad(11.5))
  Sin : Trigonometry
  Vector Concatenate : Concatenate  NumInputs=3
  m_versor : Outport
  wires:
  Clock/1 -> Gain/1
  Gain/1 -> Sin/1, Cos/1
  Gain2/1 -> Vector Concatenate/2
  Vector Concatenate/1 -> m_versor/1
  Cos/1 -> Gain1/1
  Constant/1 -> Vector Concatenate/3
  Sin/1 -> Gain2/1
  Gain1/1 -> Vector Concatenate/1

== system SAD_project/Dynamics e Kinematics/Attitude error GG/Attitude error ==
  DCM B/N : Inport
  DCM L/N : Inport  Port=2
  Matrix Multiply : Product  Multiplication=Matrix(*)
  Transpose : Math  Operator=transpose
  DCM B/L : Outport
  wires:
  Transpose/1 -> Matrix Multiply/2
  Matrix Multiply/1 -> DCM B/L/1
  DCM B/N/1 -> Matrix Multiply/1
  DCM L/N/1 -> Transpose/1

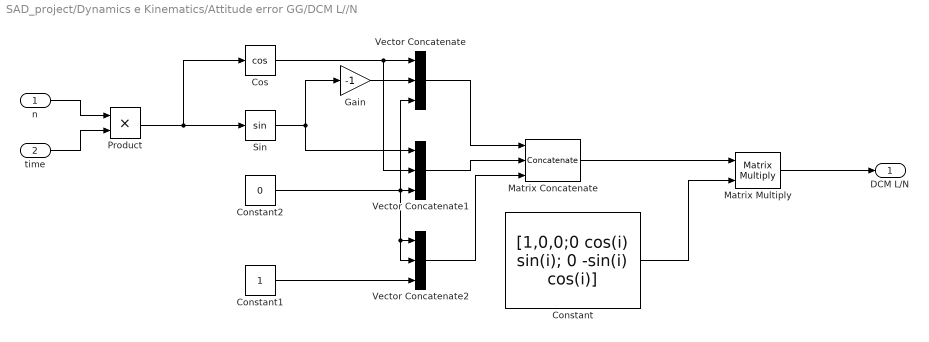
== system SAD_project/Dynamics e Kinematics/Attitude error GG/DCM L//N ==
  n : Inport
  time : Inport  Port=2
  Constant : Constant  Value=[1,0,0;0 cos(i) sin(i); 0 -sin(i) cos(i)]
  Constant1 : Constant
  Constant2 : Constant  Value=0
  Cos : Trigonometry  Operator=cos
  Gain : Gain  Gain=-1
  Matrix Concatenate : Concatenate  NumInputs=3  Mode=Multidimensional array  ConcatenateDimension=2
  Matrix Multiply : Product  Multiplication=Matrix(*)
  Product : Product
  Sin : Trigonometry
  Vector Concatenate : Concatenate  NumInputs=3
  Vector Concatenate1 : Concatenate  NumInputs=3
  Vector Concatenate2 : Concatenate  NumInputs=3
  DCM L/N : Outport
  wires:
  Product/1 -> Cos/1, Sin/1
  Gain/1 -> Vector Concatenate/2
  Vector Concatenate1/1 -> Matrix Concatenate/2
  Cos/1 -> Vector Concatenate/1, Vector Concatenate1/2
  Vector Concatenate2/1 -> Matrix Concatenate/3
  time/1 -> Product/2
  Constant2/1 -> Vector Concatenate2/1, Vector Concatenate2/2, Vector Concatenate/3, Vector Concatenate1/3
  Vector Concatenate/1 -> Matrix Concatenate/1
  Sin/1 -> Gain/1, Vector Concatenate1/1
  Constant1/1 -> Vector Concatenate2/3
  n/1 -> Product/1
  Matrix Concatenate/1 -> Matrix Multiply/1
  Constant/1 -> Matrix Multiply/2
  Matrix Multiply/1 -> DCM L/N/1

== system SAD_project/Dynamics e Kinematics/DCM composition from quaternions 1/Cross product matrix composition ==
  q_vect : Inport
  Demux : Demux  Outputs=3
  Gain : Gain  Gain=[0 0 0; 0 0 -1; 0 1 0]
  Gain1 : Gain  Gain=[0 0 1; 0 0 0; -1 0 0]
  Gain2 : Gain  Gain=[0 -1 0; 1 0 0; 0 0 0]
  Sum : Sum  Inputs=+++
  q_vect cross : Outport
  wires:
  Gain1/1 -> Sum/2
  Demux/3 -> Gain2/1
  Demux/1 -> Gain/1
  q_vect/1 -> Demux/1
  Gain2/1 -> Sum/3
  Demux/2 -> Gain1/1
  Gain/1 -> Sum/1
  Sum/1 -> q_vect cross/1

== system SAD_project/Dynamics e Kinematics/Kinematics quaternion2/Matrix OMEGA ==
  omega : Inport
  Constant4 : Constant  Value=0
  Demux : Demux  Outputs=3
  Gain : Gain  Gain=-1
  Gain1 : Gain  Gain=-1
  Gain2 : Gain  Gain=-1
  Matrix Concatenate : Concatenate  NumInputs=4  Mode=Multidimensional array  ConcatenateDimension=2
  Vector Concatenate{,2..4} (4 alike) : Concatenate  NumInputs=4
  Matrix Omega : Outport
  wires:
  Demux/2 -> Vector Concatenate4/2, Vector Concatenate/3, Gain1/1  "W_v"
  Gain1/1 -> Vector Concatenate2/4, Vector Concatenate3/1
  Matrix Concatenate/1 -> Matrix Omega/1
  Gain2/1 -> Vector Concatenate3/4, Vector Concatenate/2  "-W_w"
  Vector Concatenate3/1 -> Matrix Concatenate/3
  Demux/3 -> Vector Concatenate2/1, Vector Concatenate4/3, Gain2/1  "W_w"
  Gain/1 -> Vector Concatenate/4, Vector Concatenate2/3  "-W_u"
  Constant4/1 -> Vector Concatenate/1, Vector Concatenate2/2, Vector Concatenate3/3, Vector Concatenate4/4
  Demux/1 -> Vector Concatenate3/2, Vector Concatenate4/1, Gain/1  "W_u"
  Vector Concatenate4/1 -> Matrix Concatenate/4
  Vector Concatenate2/1 -> Matrix Concatenate/2
  Vector Concatenate/1 -> Matrix Concatenate/1
  omega/1 -> Demux/1

== system SAD_project/Dynamics e Kinematics/Kinematics quaternion2/Normalize Vector2 ==
  Vector : Inport
  Dot Product : DotProduct  OutDataTypeStr=Inherit: Inherit via internal rule
  Sqrt : Sqrt
  Norm : Outport
  wires:
  Sqrt/1 -> Norm/1
  Vector/1 -> Dot Product/1, Dot Product/2
  Dot Product/1 -> Sqrt/1

== system SAD_project/two-body Keplerian dynamics/Integretion of true anomaly/(1-e^2)^(3//2) ==
  Constant1 : Constant
  Constant2 : Constant  Value=e
  Constant3 : Constant  Value=3/2
  Power : Math  Operator=pow
  Product1 : Product
  Subtract : Sum  Inputs=+-
  Out1 : Outport
  wires:
  Constant3/1 -> Power/2
  Constant2/1 -> Product1/2, Product1/1
  Subtract/1 -> Power/1
  Constant1/1 -> Subtract/1
  Product1/1 -> Subtract/2
  Power/1 -> Out1/1

== system SAD_project/two-body Keplerian dynamics/r_perifocal/Calculation of norm r ==
  th : Inport
  Constant : Constant  Value=p
  Constant2 : Constant
  Cos : Trigonometry  Operator=cos
  Divide : Product  Inputs=*/
  Gain1 : Gain  Gain=e
  Sum : Sum  Inputs=|++
  Norm(r) : Outport
  wires:
  Constant/1 -> Divide/1
  Gain1/1 -> Sum/2
  Constant2/1 -> Sum/1
  Cos/1 -> Gain1/1
  Sum/1 -> Divide/2
  th/1 -> Cos/1
  Divide/1 -> Norm(r)/1

== system SAD_project/Calculation of disturbance torque/M of Solar Pressure/Calculation of F_i/(1-ps)*Sb + (2ps*dot(SB,Nb) +2//3pd))*Ni ==
  body : Inport
  dot(Sb,Nb) : Inport  Port=2
  Sb versor : Inport  Port=3
  Constant5 : Constant  Value=pd
  Gain1 : Gain  Gain=2*ps
  Gain2 : Gain  Gain=2/3
  Gain3 : Gain  Gain=[(A1 - ps) (A1 - ps) (A1 - ps)]
  Matrix Concatenate : Concatenate  NumInputs=3  Mode=Multidimensional array  ConcatenateDimension=2
  Matrix Muly2 : Product
  Sum : Sum  Inputs=|++
  Sum1 : Sum  Inputs=|++
  Out1 : Outport
  wires:
  Sum1/1 -> Matrix Concatenate/1, Matrix Concatenate/3, Matrix Concatenate/2  "2ps*dot(SB,Nb) +2/3pd)"
  Gain1/1 -> Sum1/1
  dot(Sb,Nb)/1 -> Gain1/1
  Gain3/1 -> Sum/2  "(1-ps)*Sb"
  Constant5/1 -> Gain2/1
  Sum/1 -> Out1/1
  Matrix Muly2/1 -> Sum/1  "(2ps*dot(SB,Nb) +2/3pd))*Ni"
  Matrix Concatenate/1 -> Matrix Muly2/2  "Sb_vector"
  Gain2/1 -> Sum1/2
  body/1 -> Matrix Muly2/1
  Sb versor/1 -> Gain3/1

== system SAD_project/Calculation of disturbance torque/M of Solar Pressure/Calculation of F_i/Eliminate effect of face in shadow ==
  dot(SB,Nb) : Inport
  Compare To Zero : simulink/Logic and Bit Operations/Compare To Zero  relop=>=  OutDataTypeStr=boolean
  Product : Product
  dot(SB,Nb)-clean : Outport
  wires:
  dot(SB,Nb)/1 -> Product/2, Compare To Zero/1
  Compare To Zero/1 -> Product/1
  Product/1 -> dot(SB,Nb)-clean/1

== system SAD_project/Calculation of disturbance torque/M of Solar Pressure/Calculation of F_i/Subsystem ==
  dot(SB,Nb) : Inport
  A : Inport  Port=2
  Gain : Gain  Gain=-Fe/c
  Product : Product
  -PA*dot(SB,Nb) : Outport
  wires:
  Product/1 -> Gain/1
  A/1 -> Product/2
  Gain/1 -> -PA*dot(SB,Nb)/1  "-PA*dot(SB,Nb)"
  dot(SB,Nb)/1 -> Product/1

== system SAD_project/Calculation of disturbance torque/M of Solar Pressure/Calculation of F_i/dot(Sb,Nb) ==
  body versor matrix : Inport
  Sb_vector1 : Inport  Port=2
  Constant2 : Constant  Value=ones(length(BODY),1)  VectorParams1D=off
  Matrix Multiply : Product  Multiplication=Matrix(*)
  Matrix Muly1 : Product
  Sum of Elements : Sum  Inputs=+  CollapseMode=Specified dimension  CollapseDim=2
  Transpose : Math  Operator=transpose
  dot(SB,Nb) : Outport
  Sb_matrix : Outport  Port=2
  wires:
  Matrix Muly1/1 -> Sum of Elements/1
  Matrix Multiply/1 -> Sb_matrix/1, Matrix Muly1/2  "Sb_vector"
  Constant2/1 -> Matrix Multiply/1
  Sb_vector1/1 -> Transpose/1
  body versor matrix/1 -> Matrix Muly1/1
  Sum of Elements/1 -> dot(SB,Nb)/1  "dot(SB,Nb)"
  Transpose/1 -> Matrix Multiply/2

== system SAD_project/Calculation of disturbance torque/M of Solar Pressure/Normalize Vector/Normalize Vector ==
  Vector : Inport
  Dot Product : DotProduct  OutDataTypeStr=Inherit: Inherit via internal rule
  Sqrt : Sqrt
  Norm : Outport
  wires:
  Sqrt/1 -> Norm/1
  Vector/1 -> Dot Product/1, Dot Product/2
  Dot Product/1 -> Sqrt/1

== system SAD_project/Calculation of disturbance torque/M of Solar Pressure/Torque calculation/Subsystem ==
  a2 : Inport
  a3 : Inport  Port=2
  Gain : Gain  Gain=r3
  Gain1 : Gain  Gain=r2
  Subtract : Sum  Inputs=+-
  M_i : Outport
  wires:
  a2/1 -> Gain/1
  a3/1 -> Gain1/1
  Gain/1 -> Subtract/1
  Gain1/1 -> Subtract/2
  Subtract/1 -> M_i/1

== system SAD_project/Calculation of disturbance torque/M of Solar Pressure/Torque calculation/Subsystem1 ==
  a3 : Inport
  a1 : Inport  Port=2
  Gain : Gain  Gain=r1
  Gain1 : Gain  Gain=r3
  Subtract : Sum  Inputs=+-
  M_j : Outport
  wires:
  a3/1 -> Gain/1
  a1/1 -> Gain1/1
  Gain/1 -> Subtract/1
  Gain1/1 -> Subtract/2
  Subtract/1 -> M_j/1

== system SAD_project/Calculation of disturbance torque/M of Solar Pressure/Torque calculation/Subsystem2 ==
  a1 : Inport
  a2 : Inport  Port=2
  Gain : Gain  Gain=r2
  Gain1 : Gain  Gain=r1
  Subtract : Sum  Inputs=+-
  M_i : Outport
  wires:
  a1/1 -> Gain/1
  a2/1 -> Gain1/1
  Gain/1 -> Subtract/1
  Gain1/1 -> Subtract/2
  Subtract/1 -> M_i/1

== system SAD_project/Dipol Model of Magnetic Field/Calculation of b_n/Normalize Vector/Normalize Vector1 ==
  Vector : Inport
  Dot Product : DotProduct  OutDataTypeStr=Inherit: Inherit via internal rule
  Sqrt : Sqrt
  Norm : Outport
  wires:
  Sqrt/1 -> Norm/1
  Vector/1 -> Dot Product/1, Dot Product/2
  Dot Product/1 -> Sqrt/1

== matlab function SAD_project/Sun Position in Earth Centred Equatorial Inertial RF/MATLAB Function1 ==
  data: MJD2000 input; r output
function r = fcn(MJD2000)
     [kep, mu_S] = uplanet(MJD2000, 3); % important that in uplanet there is an initialisation of kep like kep = zeros(6,1);
     r = kep2carRAD(kep, mu_S);
end
